simulink model "WTxPSMG"  (R2023b)
settings: Solver=ode3  StartTime=0.0  StopTime=0.1  FixedStep=0.00001  RelTol=1e-3
undefined symbols (not defined in the file): c1, c2, c3, c5, c6, J, Ke, Ld, Lq, omega_r, p, R, ro, Rs
libraries: mcbcontrolslib x6, simulink x3
settings Model: Creator=tudorn  LastModifiedBy=tudorn

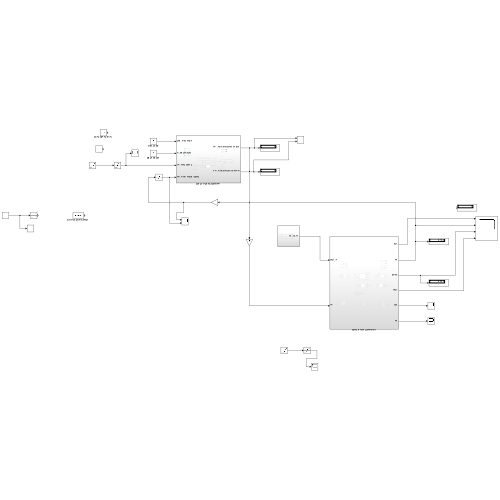
[thumbnail: Simulink's stored preview of the top-level diagram]
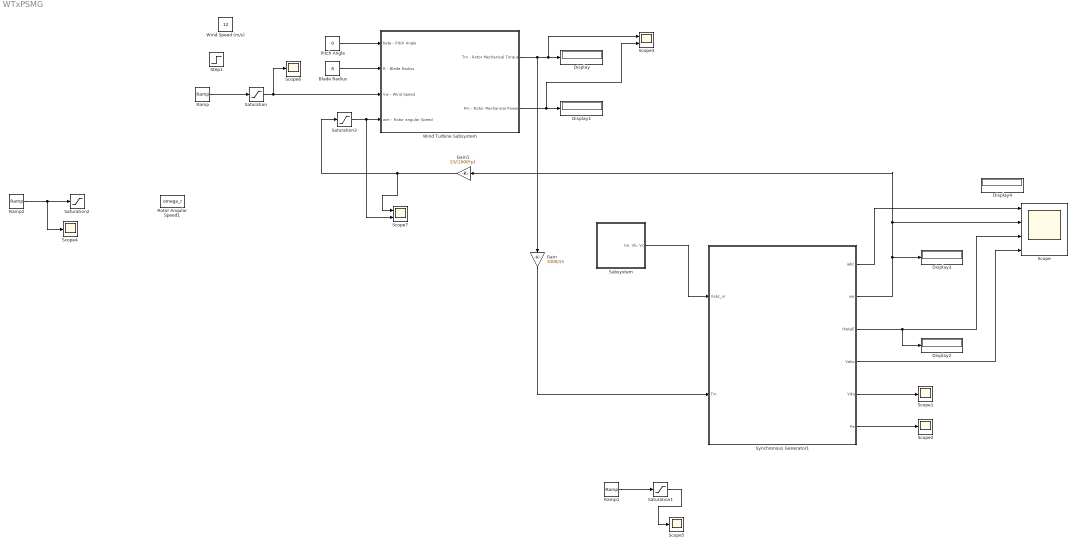
== system WTxPSMG ==
  Blade Radius : Constant  Value=R
  Display{,1..4} (5 alike) : Display
  Gain : Gain  Gain=1000/15
  Gain1 : Gain  Gain=15/(1000*p)
  Pitch Angle : Constant  Value=0
  Ramp : simulink/Sources/Ramp  slope=10  start=0.02  InitialOutput=7
  Ramp1 : simulink/Sources/Ramp  slope=1e3  start=0  InitialOutput=0
  Ramp2 : simulink/Sources/Ramp  slope=10  start=0.02  InitialOutput=0
  Rotor Angular Speed1 : Constant  Value=omega_r
  Saturation : Saturate  UpperLimit=12  LowerLimit=5
  Saturation1 : Saturate  UpperLimit=50  LowerLimit=-1
  Saturation2 : Saturate  UpperLimit=15  LowerLimit=-15
  Saturation3 : Saturate  UpperLimit=15  LowerLimit=-15
  Scope : Scope  NumInputPorts=4
  Scope{1..2,4..6} (5 alike) : Scope
  Scope3 : Scope  NumInputPorts=2
  Scope7 : Scope  NumInputPorts=2
  Step1 : Step  Time=10  Before=7  After=12  SampleTime=0
  Subsystem : Subsystem
  Synchronous Generator1 : Subsystem
  Wind Speed (m/s) : Constant  Value=12
  Wind Turbine Subsystem : Subsystem
  wires:
  Subsystem/1("Va, Vb, Vc") -> Synchronous Generator1/1(Vabc_in)
  Synchronous Generator1/6(Pe) -> Scope2/1
  Synchronous Generator1/2(we) -> Gain1/1, Scope/2, Display3/1
  Synchronous Generator1/3(thetaE) -> Display2/1, Scope/3
  Synchronous Generator1/5(Vdq) -> Scope1/1
  Synchronous Generator1/4(Vabc) -> Scope/4
  Synchronous Generator1/1(iabc) -> Scope/1
  Saturation1/1 -> Scope5/1
  Ramp1/1 -> Saturation1/1
  Pitch Angle/1 -> Wind Turbine Subsystem/1(beta - Pitch Angle)
  Blade Radius/1 -> Wind Turbine Subsystem/2(R - Blade Radius)
  Wind Turbine Subsystem/2(Pm - Rotor Mechanical Power) -> Scope3/2, Display1/1
  Wind Turbine Subsystem/1(Tm - Rotor Mechanical Torque) -> Gain/1, Scope3/1, Display/1
  Ramp/1 -> Saturation/1
  Saturation/1 -> Wind Turbine Subsystem/3(Vw - Wind Speed), Scope6/1
  Ramp2/1 -> Saturation2/1, Scope4/1
  Gain/1 -> Synchronous Generator1/2(Tm)
  Gain1/1 -> Scope7/1, Saturation3/1
  Saturation3/1 -> Scope7/2, Wind Turbine Subsystem/4(wm - Rotor angular Speed)

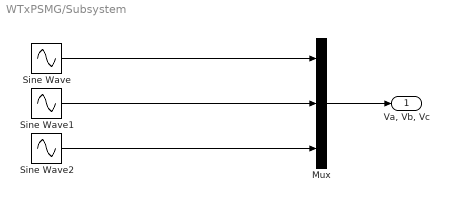
== system WTxPSMG/Subsystem ==
  Mux : Mux  Inputs=3
  Sine Wave : Sin  Amplitude=220  Frequency=2*pi*50  SampleTime=1e-5
  Sine Wave1 : Sin  Amplitude=220  Frequency=2*pi*50  Phase=2*pi/3  SampleTime=1e-5
  Sine Wave2 : Sin  Amplitude=220  Frequency=2*pi*50  Phase=-2*pi/3  SampleTime=1e-5
  "Va, Vb, Vc" : Outport
  wires:
  Mux/1 -> "Va, Vb, Vc"/1
  Sine Wave/1 -> Mux/1
  Sine Wave1/1 -> Mux/2
  Sine Wave2/1 -> Mux/3

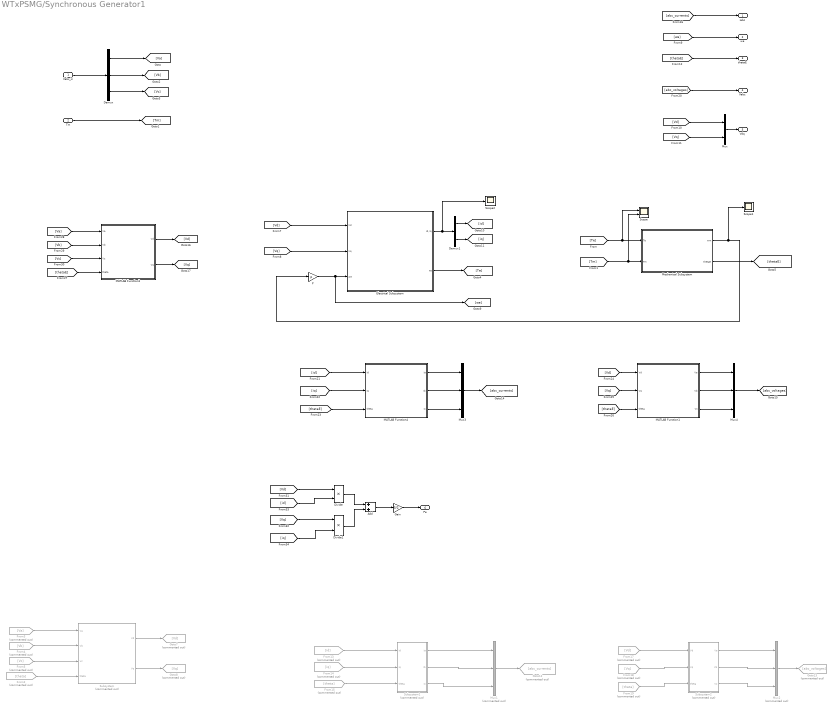
== system WTxPSMG/Synchronous Generator1 ==
  Vabc_in : Inport
  Tm : Inport  Port=2
  Add : Sum
  Demux : Demux  Outputs=3
  Demux1 : Demux  Outputs=2
  Divide : Product  Inputs=**
  Divide1 : Product  Inputs=**
  Electrical Subsystem : Subsystem
  From13 : From  Commented=on  GotoTag=id
  From14 : From  Commented=on  GotoTag=iq
  From15 : From  Commented=on  GotoTag=theta
  From17 : From  Commented=on  GotoTag=Vd
  From18 : From  Commented=on  GotoTag=Vq
  From19 : From  Commented=on  GotoTag=theta
  From2 : From  Commented=on  GotoTag=theta
  From3 : From  Commented=on  GotoTag=Va
  From4 : From  Commented=on  GotoTag=Vb
  From5 : From  Commented=on  GotoTag=Vc
  Gain : Gain  Gain=3/2
  Goto12 : Goto  Commented=on  GotoTag=abc_currents
  Goto13 : Goto  Commented=on  GotoTag=abc_voltages
  Goto7 : Goto  Commented=on  GotoTag=Vd
  Goto8 : Goto  Commented=on  GotoTag=Vq
  MATLAB Function1 : MATLAB Function  TreatAsAtomicUnit=on
  MATLAB Function3 : MATLAB Function  TreatAsAtomicUnit=on
  MATLAB Function4 : MATLAB Function  TreatAsAtomicUnit=on
  Mechanical Subsystem : Subsystem
  Mux : Mux  Inputs=2
  Mux1 : Mux  Commented=on  Inputs=3
  Mux2 : Mux  Commented=on  Inputs=3
  Mux3 : Mux  Inputs=3
  Mux4 : Mux  Inputs=3
  P : Gain  Gain=p
  Scope : Scope  NumInputPorts=2
  Scope1 : Scope
  Scope2 : Scope
  Subsystem : Subsystem  Commented=on
  Subsystem1 : Subsystem  Commented=on
  Subsystem2 : Subsystem  Commented=on
  iabc : Outport
  we : Outport  Port=2
  thetaE : Outport  Port=3
  Vabc : Outport  Port=4
  Vdq : Outport  Port=5
  Pe : Outport  Port=6
  wires:
  Vabc_in/1 -> Demux/1
  Tm/1 -> [Tm]
  Demux/1 -> [Va]
  Demux/2 -> [Vb]
  Demux/3 -> [Vc]
  Electrical Subsystem/2(Te) -> [Te]
  [Te] -> Scope/1, Mechanical Subsystem/1(Te)
  [Tm] -> Scope/2, Mechanical Subsystem/2(Tm)
  From2/1 -> Subsystem/4(theta)
  From5/1 -> Subsystem/3(Vc)
  From4/1 -> Subsystem/2(Vb)
  From3/1 -> Subsystem/1(Va)
  Mechanical Subsystem/1(wm) -> Scope1/1, P/1
  P/1 -> [we], Electrical Subsystem/3(we)
  [Vq] -> Electrical Subsystem/2(Vq)
  [Vd] -> Electrical Subsystem/1(Vd)
  Subsystem/1(Vd) -> Goto7/1
  Subsystem/2(Vq) -> Goto8/1
  [we] -> we/1
  Mux/1 -> Vdq/1
  [Vd] -> Mux/1
  [Vq] -> Mux/2
  [thetaE] -> thetaE/1
  Electrical Subsystem/1("id, iq") -> Scope2/1, Demux1/1
  Demux1/1 -> [id]
  Demux1/2 -> [iq]
  From13/1 -> Subsystem1/1(Id)
  Subsystem1/1(Ia) -> Mux1/1
  Subsystem1/3(Ic) -> Mux1/3
  Mux1/1 -> Goto12/1
  [abc_currents] -> iabc/1
  From17/1 -> Subsystem2/1(Vd)
  From18/1 -> Subsystem2/2(Vq)
  From19/1 -> Subsystem2/3(theta)
  Subsystem2/1(Va) -> Mux2/1
  Subsystem2/2(Vb) -> Mux2/2
  Subsystem2/3(Vc) -> Mux2/3
  Mux2/1 -> Goto13/1
  [abc_voltages] -> Vabc/1
  Mechanical Subsystem/2(thetaE) -> [thetaE]
  From14/1 -> Subsystem1/2(Iq)
  From15/1 -> Subsystem1/3(theta)
  Subsystem1/2(Ib) -> Mux1/2
  [iq] -> MATLAB Function4/2(Iq)
  [thetaE] -> MATLAB Function4/3(theta)
  [id] -> MATLAB Function4/1(Id)
  Mux3/1 -> [abc_currents]
  MATLAB Function4/2(Ib) -> Mux3/2
  MATLAB Function4/1(Ia) -> Mux3/1
  MATLAB Function4/3(Ic) -> Mux3/3
  [Vd] -> MATLAB Function1/1(Vd)
  [Vq] -> MATLAB Function1/2(Vq)
  [thetaE] -> MATLAB Function1/3(theta)
  Mux4/1 -> [abc_voltages]
  MATLAB Function1/1(Va) -> Mux4/1
  MATLAB Function1/2(Vb) -> Mux4/2
  MATLAB Function1/3(Vc) -> Mux4/3
  [Va] -> MATLAB Function3/1(Va)
  [Vc] -> MATLAB Function3/3(Vc)
  [thetaE] -> MATLAB Function3/4(theta)
  [Vb] -> MATLAB Function3/2(Vb)
  MATLAB Function3/2(Vq) -> [Vq]
  MATLAB Function3/1(Vd) -> [Vd]
  [Vq] -> Divide1/1
  [iq] -> Divide1/2
  [id] -> Divide/2
  [Vd] -> Divide/1
  Divide/1 -> Add/1
  Divide1/1 -> Add/2
  Add/1 -> Gain/1
  Gain/1 -> Pe/1

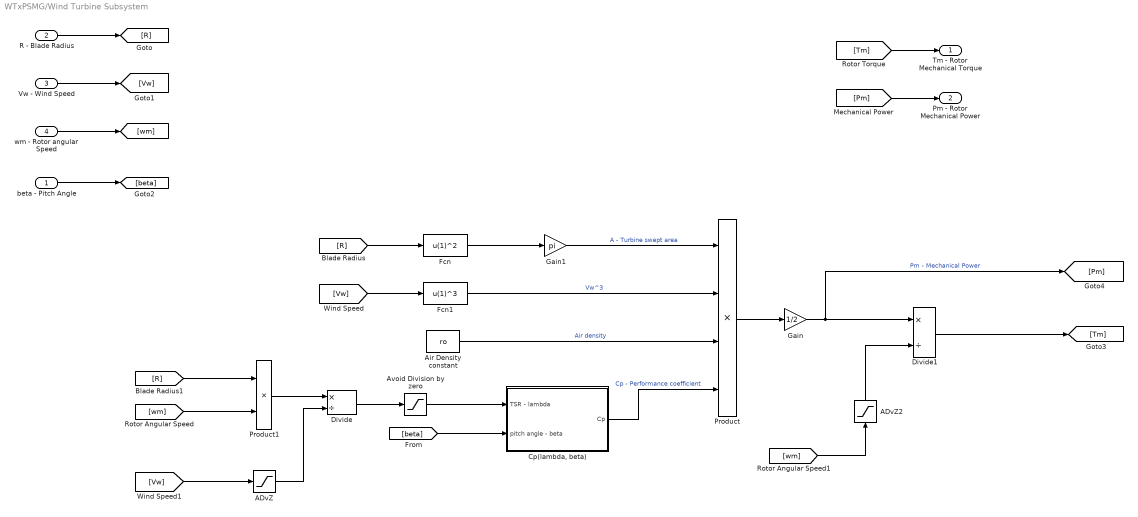
== system WTxPSMG/Wind Turbine Subsystem ==
  beta - Pitch Angle : Inport
  R - Blade Radius : Inport  Port=2
  Vw - Wind Speed : Inport  Port=3
  wm - Rotor angular Speed : Inport  Port=4
  ADvZ : Saturate  UpperLimit=1e6  LowerLimit=1e-6
  ADvZ2 : Saturate  UpperLimit=omega_r  LowerLimit=1e-6
  Air Density constant : Constant  Value=ro
  Avoid Division by zero : Saturate  UpperLimit=Inf  LowerLimit=1e-6
  "Cp(lambda, beta)" : Subsystem
  Divide : Product  Inputs=*/
  Divide1 : Product  Inputs=*/
  Fcn : Fcn  Expr=u(1)^2
  Fcn1 : Fcn  Expr=u(1)^3
  Gain : Gain  Gain=1/2
  Gain1 : Gain  Gain=pi
  Product : Product  Inputs=4
  Product1 : Product
  Tm - Rotor Mechanical Torque : Outport
  Pm - Rotor Mechanical Power : Outport  Port=2
  wires:
  Product/1 -> Gain/1
  Gain1/1 -> Product/1  "A - Turbine swept area"
  Fcn1/1 -> Product/2  "Vw^3"
  Air Density constant/1 -> Product/3  "Air density"
  "Cp(lambda, beta)"/1(Cp) -> Product/4  "Cp - Performance coefficient"
  Fcn/1 -> Gain1/1
  R - Blade Radius/1 -> [R]
  Vw - Wind Speed/1 -> [Vw]
  [R] -> Fcn/1
  [Vw] -> Fcn1/1
  wm - Rotor angular Speed/1 -> [wm]
  [R] -> Product1/1
  [wm] -> Product1/2
  Product1/1 -> Divide/1
  [Vw] -> ADvZ/1
  Divide/1 -> Avoid Division by zero/1
  ADvZ/1 -> Divide/2
  beta - Pitch Angle/1 -> [beta]
  [beta] -> "Cp(lambda, beta)"/2(pitch angle - beta)
  [Tm] -> Tm - Rotor Mechanical Torque/1
  Gain/1 -> Divide1/1, [Pm]  "Pm - Mechanical Power"
  [wm] -> ADvZ2/1
  [Pm] -> Pm - Rotor Mechanical Power/1
  ADvZ2/1 -> Divide1/2
  Avoid Division by zero/1 -> "Cp(lambda, beta)"/1(TSR - lambda)
  Divide1/1 -> [Tm]

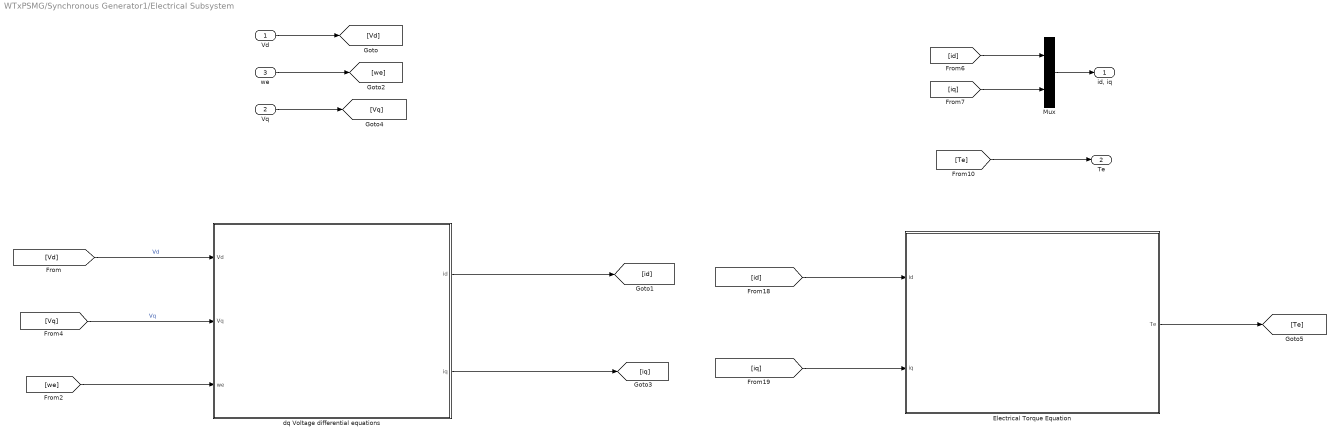
== system WTxPSMG/Synchronous Generator1/Electrical Subsystem ==
  Vd : Inport
  Vq : Inport  Port=2
  we : Inport  Port=3
  Electrical Torque Equation : Subsystem
  Mux : Mux  Inputs=2
  dq Voltage differential equations : Subsystem
  "id, iq" : Outport
  Te : Outport  Port=2
  wires:
  Vd/1 -> [Vd]
  we/1 -> [we]
  Vq/1 -> [Vq]
  Mux/1 -> "id, iq"/1
  [id] -> Mux/1
  [iq] -> Mux/2
  [Te] -> Te/1
  [Vd] -> dq Voltage differential equations/1(Vd)  "Vd"
  [Vq] -> dq Voltage differential equations/2(Vq)  "Vq"
  dq Voltage differential equations/1(id) -> [id]
  dq Voltage differential equations/2(iq) -> [iq]
  [id] -> Electrical Torque Equation/1(id)
  [iq] -> Electrical Torque Equation/2(iq)
  Electrical Torque Equation/1(Te) -> [Te]
  [we] -> dq Voltage differential equations/3(we)

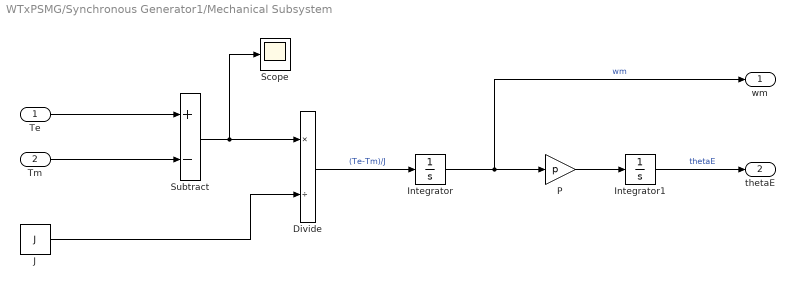
== system WTxPSMG/Synchronous Generator1/Mechanical Subsystem ==
  Te : Inport
  Tm : Inport  Port=2
  Divide : Product  Inputs=*/
  Integrator : Integrator
  Integrator1 : Integrator
  J : Constant  Value=J
  P : Gain  Gain=p
  Scope : Scope
  Subtract : Sum  Inputs=+-
  wm : Outport
  thetaE : Outport  Port=2
  wires:
  Tm/1 -> Subtract/2
  Te/1 -> Subtract/1
  Subtract/1 -> Scope/1, Divide/1
  J/1 -> Divide/2
  Divide/1 -> Integrator/1  "(Te-Tm)/J"
  Integrator/1 -> P/1, wm/1  "wm"
  Integrator1/1 -> thetaE/1  "thetaE"
  P/1 -> Integrator1/1

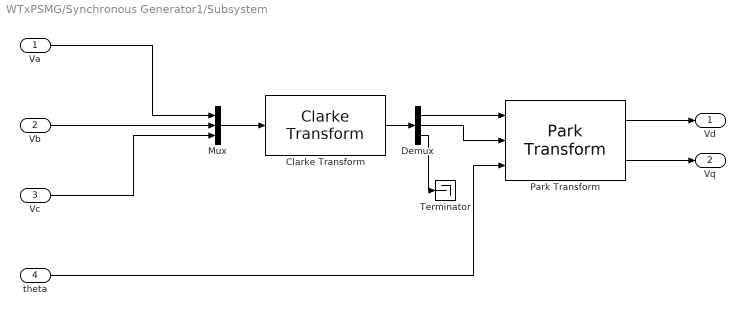
== system WTxPSMG/Synchronous Generator1/Subsystem ==
  Va : Inport
  Vb : Inport  Port=2
  Vc : Inport  Port=3
  theta : Inport  Port=4
  Clarke Transform : mcbcontrolslib/Clarke Transform  VariantControl=Variant2  PhaseInput=Three inputs  EnPowerInv=off
      settings: LibrarySourceBlock=mcbhdllib/Controls/Math Transforms/Clarke Transform
  Demux : Demux  Outputs=3
  Mux : Mux  Inputs=3
  Park Transform : mcbcontrolslib/Park Transform  PhaseInput=Two inputs  AxisAlignment=D-axis  ThetaInput=Electrical position  AngleInput=Radians  N_points=1024
      settings: LibrarySourceBlock=mcbhdllib/Controls/Math Transforms/Park Transform
  Terminator : Terminator
  Vd : Outport
  Vq : Outport  Port=2
  wires:
  Park Transform/1 -> Vd/1
  Park Transform/2 -> Vq/1
  theta/1 -> Park Transform/3
  Mux/1 -> Clarke Transform/1
  Vc/1 -> Mux/3
  Va/1 -> Mux/1
  Vb/1 -> Mux/2
  Clarke Transform/1 -> Demux/1
  Demux/1 -> Park Transform/1
  Demux/2 -> Park Transform/2
  Demux/3 -> Terminator/1

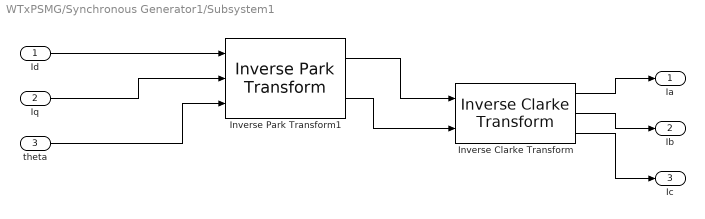
== system WTxPSMG/Synchronous Generator1/Subsystem1 ==
  Id : Inport
  Iq : Inport  Port=2
  theta : Inport  Port=3
  Inverse Clarke Transform : mcbcontrolslib/Inverse Clarke Transform  PhaseInput=Two inputs  EnPowerInv=off
      settings: LibrarySourceBlock=mcbhdllib/Controls/Math Transforms/Inverse Clarke Transform
  Inverse Park Transform1 : mcbcontrolslib/Inverse Park Transform  PhaseInput=Two inputs  AxisAlignment=D-axis  ThetaInput=Electrical position  AngleInput=Radians  N_points=1024
      settings: LibrarySourceBlock=mcbhdllib/Controls/Math Transforms/Inverse Park Transform
  Ia : Outport
  Ib : Outport  Port=2
  Ic : Outport  Port=3
  wires:
  Id/1 -> Inverse Park Transform1/1
  Iq/1 -> Inverse Park Transform1/2
  theta/1 -> Inverse Park Transform1/3
  Inverse Park Transform1/1 -> Inverse Clarke Transform/1
  Inverse Park Transform1/2 -> Inverse Clarke Transform/2
  Inverse Clarke Transform/1 -> Ia/1
  Inverse Clarke Transform/2 -> Ib/1
  Inverse Clarke Transform/3 -> Ic/1

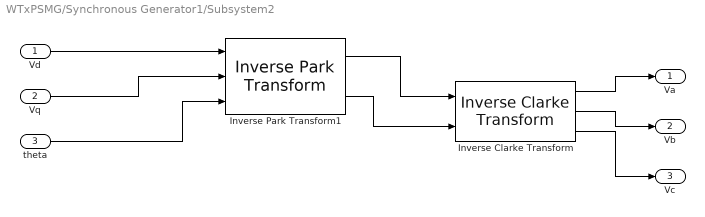
== system WTxPSMG/Synchronous Generator1/Subsystem2 ==
  Vd : Inport
  Vq : Inport  Port=2
  theta : Inport  Port=3
  Inverse Clarke Transform : mcbcontrolslib/Inverse Clarke Transform  PhaseInput=Two inputs  EnPowerInv=off
      settings: LibrarySourceBlock=mcbhdllib/Controls/Math Transforms/Inverse Clarke Transform
  Inverse Park Transform1 : mcbcontrolslib/Inverse Park Transform  PhaseInput=Two inputs  AxisAlignment=D-axis  ThetaInput=Electrical position  AngleInput=Radians  N_points=1024
      settings: LibrarySourceBlock=mcblib/Controls/Math Transforms/Inverse Park Transform
  Va : Outport
  Vb : Outport  Port=2
  Vc : Outport  Port=3
  wires:
  Vd/1 -> Inverse Park Transform1/1
  Vq/1 -> Inverse Park Transform1/2
  theta/1 -> Inverse Park Transform1/3
  Inverse Park Transform1/1 -> Inverse Clarke Transform/1
  Inverse Park Transform1/2 -> Inverse Clarke Transform/2
  Inverse Clarke Transform/1 -> Va/1
  Inverse Clarke Transform/2 -> Vb/1
  Inverse Clarke Transform/3 -> Vc/1

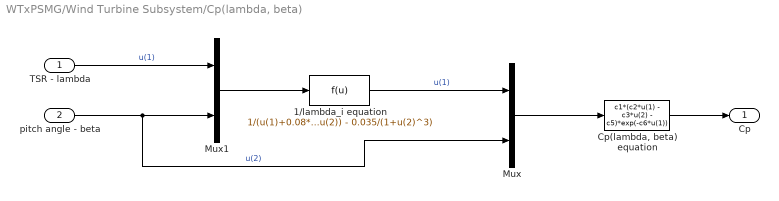
== system WTxPSMG/Wind Turbine Subsystem/Cp(lambda, beta) ==
  TSR - lambda : Inport
  pitch angle - beta : Inport  Port=2
  1/lambda_i equation : Fcn  Expr=1/(u(1)+0.08*u(2)) - 0.035/(1+u(2)^3)
  "Cp(lambda, beta) equation" : Fcn  Expr=c1*(c2*u(1) - c3*u(2) - c5)*exp(-c6*u(1))
  Mux : Mux  Inputs=2
  Mux1 : Mux  Inputs=2
  Cp : Outport
  wires:
  "Cp(lambda, beta) equation"/1 -> Cp/1
  Mux/1 -> "Cp(lambda, beta) equation"/1
  1/lambda_i equation/1 -> Mux/1  "u(1)"
  pitch angle - beta/1 -> Mux/2, Mux1/2  "u(2)"
  Mux1/1 -> 1/lambda_i equation/1
  TSR - lambda/1 -> Mux1/1  "u(1)"

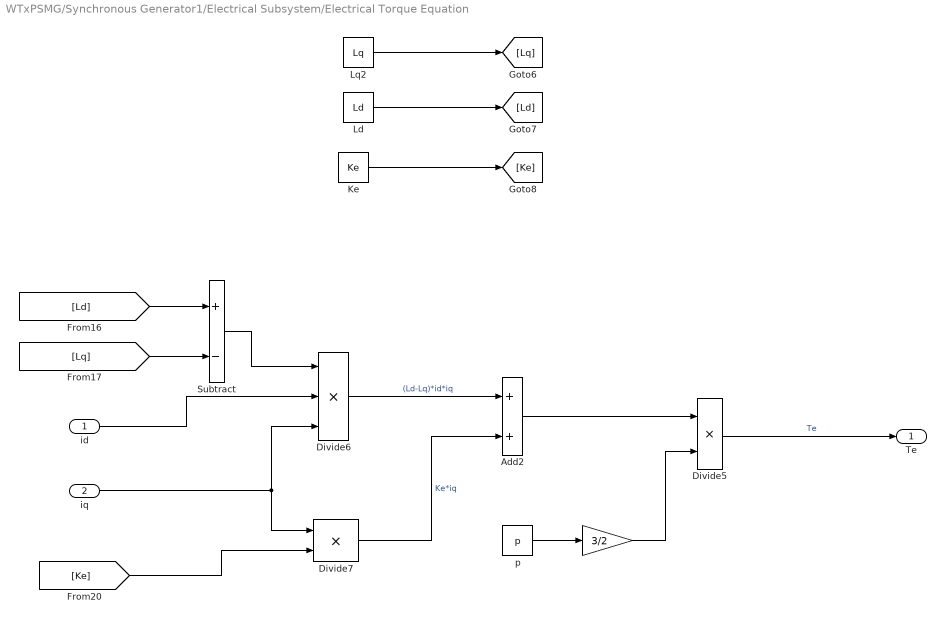
== system WTxPSMG/Synchronous Generator1/Electrical Subsystem/Electrical Torque Equation ==
  id : Inport
  iq : Inport  Port=2
  " " : Gain  Gain=3/2
  Add2 : Sum
  Divide5 : Product  Inputs=**
  Divide6 : Product  Inputs=***
  Divide7 : Product  Inputs=**
  Ke : Constant  Value=Ke
  Ld : Constant  Value=Ld
  Lq2 : Constant  Value=Lq
  Subtract : Sum  Inputs=+-
  p : Constant  Value=p
  Te : Outport
  wires:
  id/1 -> Divide6/2
  [Ke] -> Divide7/2
  Divide5/1 -> Te/1  "Te"
  " "/1 -> Divide5/2
  iq/1 -> Divide7/1, Divide6/3
  [Ld] -> Subtract/1
  Subtract/1 -> Divide6/1
  p/1 -> " "/1
  Add2/1 -> Divide5/1
  Divide6/1 -> Add2/1  "(Ld-Lq)*id*iq"
  [Lq] -> Subtract/2
  Divide7/1 -> Add2/2  "Ke*iq"
  Ld/1 -> [Ld]
  Lq2/1 -> [Lq]
  Ke/1 -> [Ke]

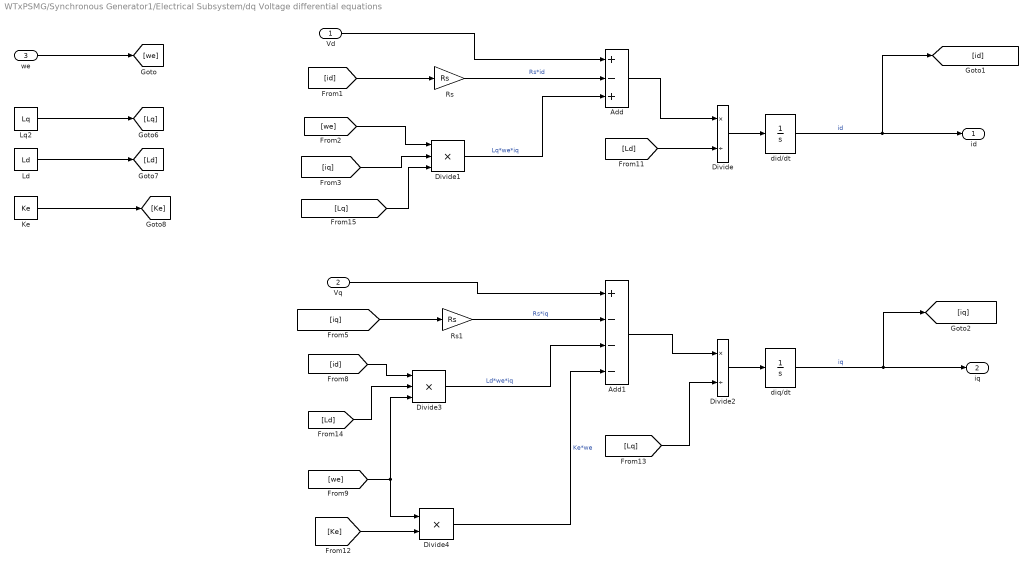
== system WTxPSMG/Synchronous Generator1/Electrical Subsystem/dq Voltage differential equations ==
  Vd : Inport
  Vq : Inport  Port=2
  we : Inport  Port=3
  Add : Sum  Inputs=+-+
  Add1 : Sum  Inputs=+---
  Divide : Product  Inputs=*/
  Divide1 : Product  Inputs=***
  Divide2 : Product  Inputs=*/
  Divide3 : Product  Inputs=***
  Divide4 : Product  Inputs=**
  Ke : Constant  Value=Ke
  Ld : Constant  Value=Ld
  Lq2 : Constant  Value=Lq
  Rs : Gain  Gain=Rs
  Rs1 : Gain  Gain=Rs
  did/dt : Integrator
  diq/dt : Integrator
  id : Outport
  iq : Outport  Port=2
  wires:
  diq/dt/1 -> [iq], iq/1  "iq"
  Add/1 -> Divide/1
  did/dt/1 -> [id], id/1  "id"
  Rs1/1 -> Add1/2  "Rs*iq"
  [Lq] -> Divide2/2
  Vq/1 -> Add1/1
  [iq] -> Divide1/2
  [id] -> Divide3/1
  Divide1/1 -> Add/3  "Lq*we*iq"
  Add1/1 -> Divide2/1
  [iq] -> Rs1/1
  [Ld] -> Divide3/2
  Divide2/1 -> diq/dt/1
  [Lq] -> Divide1/3
  Rs/1 -> Add/2  "Rs*id"
  [we] -> Divide1/1
  Divide/1 -> did/dt/1
  [Ke] -> Divide4/2
  [we] -> Divide3/3, Divide4/1
  Divide4/1 -> Add1/4  "Ke*we"
  Divide3/1 -> Add1/3  "Ld*we*iq"
  [id] -> Rs/1
  Vd/1 -> Add/1
  [Ld] -> Divide/2
  Ld/1 -> [Ld]
  Lq2/1 -> [Lq]
  Ke/1 -> [Ke]
  we/1 -> [we]

== matlab function WTxPSMG/Synchronous Generator1/MATLAB Function1 ==
  data: Vd input; Va output; Vq input; theta input; Vb output; Vc output
function [Va, Vb, Vc] = Inverse_ClarkePark_Voltage(Vd, Vq, theta)

    if isempty(theta)
        theta = 0;
    end

    Valpha = Vd .* cos(theta) - Vq .* sin(theta);
    Vbeta = Vd .* sin(theta) + Vq .* cos(theta);

    Va = Valpha;
    Vb = Valpha * (-1)/2 + Vbeta * sqrt(3)/2;
    Vc = Valpha * (-1)/2 - Vbeta * sqrt(3)/2;



end

== matlab function WTxPSMG/Synchronous Generator1/MATLAB Function3 ==
  data: Va input; Vd output; Vb input; Vc input; theta input; Vq output
function [Vd, Vq] = ClarkePark(Va, Vb, Vc, theta)

    if isempty(theta)
        theta = 0;
    end
    
    Valpha = 2/3 * (Va - 0.5 * Vb - 0.5 * Vc);
    Vbeta = 2/3 * (sqrt(3)/2 * Vb - sqrt(3)/2 * Vc);

    Vd = Valpha .* cos(theta) + Vbeta .* sin(theta);
    Vq = -Valpha .* sin(theta) + Vbeta .* cos(theta);

end

== matlab function WTxPSMG/Synchronous Generator1/MATLAB Function4 ==
  data: Id input; Ia output; Iq input; theta input; Ib output; Ic output
function [Ia, Ib, Ic] = Inverse_ClarkePark_Current(Id, Iq, theta)

    if isempty(theta)
        theta = 0;
    end

    Ialpha = Id .* cos(theta) - Iq .* sin(theta);
    Ibeta = Id .* sin(theta) + Iq .* cos(theta);

    Ia = Ialpha;
    Ib = Ialpha * (-1)/2 + Ibeta * sqrt(3)/2;
    Ic = Ialpha * (-1)/2 - Ibeta * sqrt(3)/2;


end
